simulink model "controlMCUSlugsMKIINewNav"  (Simulink 7.8)
settings: Solver=FixedStepDiscrete  SolverMode=SingleTasking  StartTime=0.0  StopTime=inf  FixedStep=0.01  RelTol=1e-3
InitFcn:
  | mcuInit
values from neighbouring files (symbols this model uses):
  apSampleTime = 0.01    [mcuInit.m]
  T = 0.01    [mcuInit.m]
undefined symbols (not defined in the file or in its folder): bda, bde, bdr, bdt, bICda, bICde, bICdr, bICdt, bpan, bPWMpan, bPWMtilt, broll, btilt, changeZoom, controlMCUInit, daTrimMax, daTrimMin, deTrimMax, deTrimMin, drTrimMax, drTrimMin, dtTrimMax, dtTrimMin, Function_Update, getAccBias, getAccels, getAttitude, getGSLocation, getISRLocation, getMidLevelCommands, getMobileLocation, getPassValues, getRangeOfParams, getRTB, getVned, getXYZ, gsRead, Init_onlyOnce, Init_Reset, mda, mde, mdr, mdt, mICda, mICde, mICdr, mICdt, mpan, mPWMpan, mPWMtilt, mroll, mtilt, PAR_CAM_X, PAR_CAM_Z, PAR_CONFIG_ROLL_R, PAR_CONFIG_YAW_R, PAR_L1_OMEGA, PAR_L1_ON_OFF, PAR_NAV_ISR_FAC, PAR_NAV_L2_BASE ... (+34)
libraries: dsPICdrivers x84, SLUGS_Library x12, simulink x7, aerolibobsolete x3, aerolibconvert2 x3, dspmtrx3 x1, aerolibtransform2 x1
(part 2 of 4)

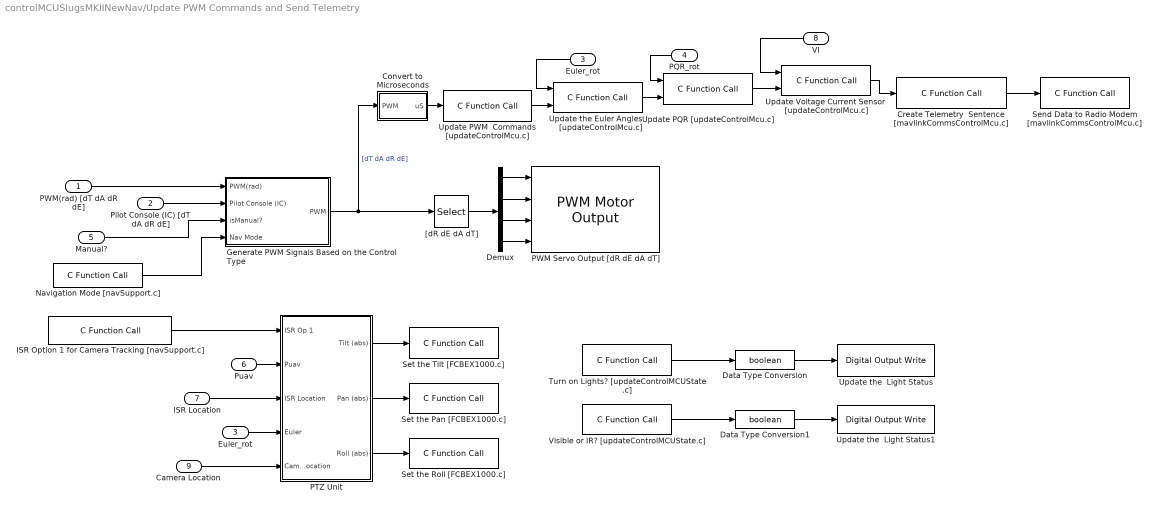
== system controlMCUSlugsMKIINewNav/Update PWM Commands and Send Telemetry ==
  PWM(rad) [dT dA dR dE] : Inport
  Pilot Console (IC) [dT dA dR dE] : Inport  Port=2
  Euler_rot : Inport  Port=3
  PQR_rot : Inport  Port=4
  Manual? : Inport  Port=5
  Puav : Inport  Port=6
  ISR Location : Inport  Port=7
  VI : Inport  Port=8
  Camera Location : Inport  Port=9
  Convert to Microseconds : Subsystem
  Create Telemetry  Sentence [mavlinkCommsControlMcu.c] : dsPICdrivers/OTHERS/C Function Call  Tag=dsPIC_dsPIC_CFunctionCall  FctUpdate=Output Function  fctName='prepareTelemetryMavlink'  INPUT_SIZE=1  INPUT1=--  INPUT2=--  INPUT3=--  OUTPUT_SIZE=120  OUTPUT1=uint8  SampleTime=.02  InputType=[ ]  OutputType=[ 2 ]  FctDeclaration=extern void prepareTelemetryMavlink(uint8_T* y1);  FctCall=prepareTelemetryMavlink(*%y1);  OrderingInOutPopup=Input  FctStart=None  FctStart_Name=Init_onlyOnce  FctStart_Declaration=inline extern void Init_onlyOnce();  FctStart_Call=Init_onlyOnce();  FctInit=None  FctInit_Name=Init_Reset  FctInit_Declaration=inline extern void Init_Reset();  FctInit_Call=Init_Reset();  PinDigitalInput=[]  PinDigitalOutput=[]  AnalogueInput=[]
  Data Type Conversion : DataTypeConversion  OutDataTypeStr=boolean
  Data Type Conversion1 : DataTypeConversion  OutDataTypeStr=boolean
  Demux : Demux
  "Euler_rot " : InportShadow  Port=3
  Generate PWM Signals Based on the Control Type : Subsystem
  ISR Option 1 for Camera Tracking [navSupport.c] : dsPICdrivers/OTHERS/C Function Call  Tag=dsPIC_dsPIC_CFunctionCall  FctUpdate=Output Function  fctName='getISRCameraOption1'  INPUT_SIZE=1  INPUT1=--  INPUT2=--  INPUT3=--  OUTPUT_SIZE=1  OUTPUT1=uint8  SampleTime=.01  InputType=[ ]  OutputType=[ 2 ]  FctDeclaration=extern uint8_T getISRCameraOption1();  FctCall=%y1 = getISRCameraOption1();  OrderingInOutPopup=None  FctStart=None  FctStart_Name=Init_onlyOnce  FctStart_Declaration=inline extern void Init_onlyOnce();  FctStart_Call=Init_onlyOnce();  FctInit=None  FctInit_Name=Init_Reset  FctInit_Declaration=inline extern void Init_Reset();  FctInit_Call=Init_Reset();  PinDigitalInput=[]  PinDigitalOutput=[]  AnalogueInput=[]
  Navigation Mode [navSupport.c] : dsPICdrivers/OTHERS/C Function Call  Tag=dsPIC_dsPIC_CFunctionCall  FctUpdate=Output Function  fctName='getNavMode'  INPUT_SIZE=1  INPUT1=--  INPUT2=--  INPUT3=--  OUTPUT_SIZE=1  OUTPUT1=uint8  SampleTime=.01  InputType=[ ]  OutputType=[ 2 ]  FctDeclaration=extern uint8_T getNavMode();  FctCall=%y1 = getNavMode();  OrderingInOutPopup=None  FctStart=None  FctStart_Name=Init_onlyOnce  FctStart_Declaration=inline extern void Init_onlyOnce();  FctStart_Call=Init_onlyOnce();  FctInit=None  FctInit_Name=Init_Reset  FctInit_Declaration=inline extern void Init_Reset();  FctInit_Call=Init_Reset();  PinDigitalInput=[]  PinDigitalOutput=[]  AnalogueInput=[]
  PTZ Unit : Subsystem
  PWM Servo Output [dR dE dA dT] : dsPICdrivers/Peripheral I//O/PWM Motor Output  Tag=dsPIC_PWM_Motor  Priority=5  PWMref=1  PWM12=1  InputEnableChk=off  InputPeriodeChk=off  Channel=[1 2 3 4]  TPeriode=.02  PrescalerValue=16  PeriodeInteger=25000  MaxName='PWM'  Centered=on  HChannelON=off  Info="Nbr Bits : 15.6096  ||  PWM = 50000  ||  Prescaler = 16"  Delay=0  IntPriority=5  nbrPwmChannelPIC=4  Status=OK  DeadTimePrescaleA=.0126*1e-3  DeadTimePrescaleB=0  DeadTimeInfo="Dead Time A = 1.26e-005  ||  Dead Time B = 0"  DTPWM1a=Prescaler A  DTPWM1i=Prescaler A  DTPWM2a=Prescaler A  DTPWM2i=Prescaler A  DTPWM3a=Prescaler A  DTPWM3i=Prescaler A  DTPWM4a=Prescaler A  DTPWM4i=Prescaler A  DTCON1=255  DTCON2=0  FAULTA_FLATM=Re-Enable PWM when Fault Pin is desactivated  FaultA_Output=off  FaultA_PWM1_State=No Changes (PWM)  FaultA_PWM2_State=No Changes (PWM)  FaultA_PWM3_State=No Changes (PWM)  FaultA_PWM4_State=No Changes (PWM)  OVDCON=off
  Send Data to Radio Modem [mavlinkCommsControlMcu.c] : dsPICdrivers/OTHERS/C Function Call  Tag=dsPIC_dsPIC_CFunctionCall  FctUpdate=Output Function  fctName='send2GS'  INPUT_SIZE=120  INPUT1=uint8  INPUT2=--  INPUT3=--  OUTPUT_SIZE=1  OUTPUT1=--  SampleTime=0.02  InputType=[ 2 ]  OutputType=[ ]  FctDeclaration=extern void send2GS(uint8_T* u1);  FctCall=send2GS(*%u1);  OrderingInOutPopup=None  FctStart=None  FctStart_Name=Init_onlyOnce  FctStart_Declaration=inline extern void Init_onlyOnce();  FctStart_Call=Init_onlyOnce();  FctInit=None  FctInit_Name=Init_Reset  FctInit_Declaration=inline extern void Init_Reset();  FctInit_Call=Init_Reset();  PinDigitalInput=[]  PinDigitalOutput=[]  AnalogueInput=[]
  Set the Pan [FCBEX1000.c] : dsPICdrivers/OTHERS/C Function Call  Tag=dsPIC_dsPIC_CFunctionCall  FctUpdate=Output Function  fctName='updatePan'  INPUT_SIZE=1  INPUT1=uint16  INPUT2=--  INPUT3=--  OUTPUT_SIZE=1  OUTPUT1=--  SampleTime=-1  InputType=[ 4 ]  OutputType=[ ]  FctDeclaration=extern void updatePan(uint16_T u1);  FctCall=updatePan(%u1);  OrderingInOutPopup=None  FctStart=None  FctStart_Name=Init_onlyOnce  FctStart_Declaration=inline extern void Init_onlyOnce();  FctStart_Call=Init_onlyOnce();  FctInit=None  FctInit_Name=Init_Reset  FctInit_Declaration=inline extern void Init_Reset();  FctInit_Call=Init_Reset();  PinDigitalInput=[]  PinDigitalOutput=[]  AnalogueInput=[]
  Set the Roll [FCBEX1000.c] : dsPICdrivers/OTHERS/C Function Call  Tag=dsPIC_dsPIC_CFunctionCall  FctUpdate=Output Function  fctName='updateRoll'  INPUT_SIZE=1  INPUT1=uint16  INPUT2=--  INPUT3=--  OUTPUT_SIZE=1  OUTPUT1=--  SampleTime=-1  InputType=[ 4 ]  OutputType=[ ]  FctDeclaration=extern void updateRoll(uint16_T u1);  FctCall=updateRoll(%u1);  OrderingInOutPopup=None  FctStart=None  FctStart_Name=Init_onlyOnce  FctStart_Declaration=inline extern void Init_onlyOnce();  FctStart_Call=Init_onlyOnce();  FctInit=None  FctInit_Name=Init_Reset  FctInit_Declaration=inline extern void Init_Reset();  FctInit_Call=Init_Reset();  PinDigitalInput=[]  PinDigitalOutput=[]  AnalogueInput=[]
  Set the Tilt [FCBEX1000.c] : dsPICdrivers/OTHERS/C Function Call  Tag=dsPIC_dsPIC_CFunctionCall  FctUpdate=Output Function  fctName='updateTilt'  INPUT_SIZE=1  INPUT1=uint16  INPUT2=--  INPUT3=--  OUTPUT_SIZE=1  OUTPUT1=--  SampleTime=-1  InputType=[ 4 ]  OutputType=[ ]  FctDeclaration=extern void updateTilt(uint16_T u1);  FctCall=updateTilt(%u1);  OrderingInOutPopup=None  FctStart=None  FctStart_Name=Init_onlyOnce  FctStart_Declaration=inline extern void Init_onlyOnce();  FctStart_Call=Init_onlyOnce();  FctInit=None  FctInit_Name=Init_Reset  FctInit_Declaration=inline extern void Init_Reset();  FctInit_Call=Init_Reset();  PinDigitalInput=[]  PinDigitalOutput=[]  AnalogueInput=[]
  Turn on Lights? [updateControlMCUState.c] : dsPICdrivers/OTHERS/C Function Call  Tag=dsPIC_dsPIC_CFunctionCall  FctUpdate=Output Function  fctName='getLightsOnOff'  INPUT_SIZE=1  INPUT1=--  INPUT2=--  INPUT3=--  OUTPUT_SIZE=1  OUTPUT1=uint8  SampleTime=0.01  InputType=[ ]  OutputType=[ 2 ]  FctDeclaration=extern uint8_T getLightsOnOff();  FctCall=%y1 = getLightsOnOff();  OrderingInOutPopup=None  FctStart=None  FctStart_Name=Init_onlyOnce  FctStart_Declaration=inline extern void Init_onlyOnce();  FctStart_Call=Init_onlyOnce();  FctInit=None  FctInit_Name=Init_Reset  FctInit_Declaration=inline extern void Init_Reset();  FctInit_Call=Init_Reset();  PinDigitalInput=[]  PinDigitalOutput=[]  AnalogueInput=[]
  "Update PQR [updateControlMcu.c] " : dsPICdrivers/OTHERS/C Function Call  Tag=dsPIC_dsPIC_CFunctionCall  FctUpdate=Output Function  fctName='updatePQR'  INPUT_SIZE=3  INPUT1=real32  INPUT2=--  INPUT3=--  OUTPUT_SIZE=1  OUTPUT1=--  SampleTime=.01  InputType=[ 7 ]  OutputType=[ ]  FctDeclaration=extern void updatePQR(real32_T* u1);  FctCall=updatePQR(*%u1);  OrderingInOutPopup=Input & Output  FctStart=None  FctStart_Name=Init_onlyOnce  FctStart_Declaration=inline extern void Init_onlyOnce();  FctStart_Call=Init_onlyOnce();  FctInit=None  FctInit_Name=Init_Reset  FctInit_Declaration=inline extern void Init_Reset();  FctInit_Call=Init_Reset();  PinDigitalInput=[]  PinDigitalOutput=[]  AnalogueInput=[]
  Update PWM  Commands [updateControlMcu.c] : dsPICdrivers/OTHERS/C Function Call  Tag=dsPIC_dsPIC_CFunctionCall  FctUpdate=Output Function  fctName='updatePWM'  INPUT_SIZE=4  INPUT1=uint16  INPUT2=--  INPUT3=--  OUTPUT_SIZE=1  OUTPUT1=--  SampleTime=-1  InputType=[ 4 ]  OutputType=[ ]  FctDeclaration=extern void updatePWM(uint16_T* u1);  FctCall=updatePWM(*%u1);  OrderingInOutPopup=Output  FctStart=None  FctStart_Name=Init_onlyOnce  FctStart_Declaration=inline extern void Init_onlyOnce();  FctStart_Call=Init_onlyOnce();  FctInit=None  FctInit_Name=Init_Reset  FctInit_Declaration=inline extern void Init_Reset();  FctInit_Call=Init_Reset();  PinDigitalInput=[]  PinDigitalOutput=[]  AnalogueInput=[]
  Update Voltage Current Sensor  [updateControlMcu.c] : dsPICdrivers/OTHERS/C Function Call  Tag=dsPIC_dsPIC_CFunctionCall  FctUpdate=Output Function  fctName='updateVISensor'  INPUT_SIZE=2  INPUT1=uint16  INPUT2=--  INPUT3=--  OUTPUT_SIZE=1  OUTPUT1=--  SampleTime=.01  InputType=[ 4 ]  OutputType=[ ]  FctDeclaration=extern void updateVISensor(uint16_T* u1);  FctCall=updateVISensor(*%u1);  OrderingInOutPopup=Input & Output  FctStart=None  FctStart_Name=Init_onlyOnce  FctStart_Declaration=inline extern void Init_onlyOnce();  FctStart_Call=Init_onlyOnce();  FctInit=None  FctInit_Name=Init_Reset  FctInit_Declaration=inline extern void Init_Reset();  FctInit_Call=Init_Reset();  PinDigitalInput=[]  PinDigitalOutput=[]  AnalogueInput=[]
  Update the  Light Status : dsPICdrivers/Digital I//O/Digital Output Write  Tag=dsPIC_Digital_Output  Priority=5  PORT=G  Pin=[15]  Simultaneous=off  OrderingInOutPopup=None
  Update the  Light Status1 : dsPICdrivers/Digital I//O/Digital Output Write  Tag=dsPIC_Digital_Output  Priority=5  PORT=G  Pin=[7]  Simultaneous=off  OrderingInOutPopup=None
  "Update the Euler Angles [updateControlMcu.c] " : dsPICdrivers/OTHERS/C Function Call  Tag=dsPIC_dsPIC_CFunctionCall  FctUpdate=Output Function  fctName='updateEuler'  INPUT_SIZE=3  INPUT1=real32  INPUT2=--  INPUT3=--  OUTPUT_SIZE=1  OUTPUT1=--  SampleTime=.01  InputType=[ 7 ]  OutputType=[ ]  FctDeclaration=extern void updateEuler(real32_T* u1);  FctCall=updateEuler(*%u1);  OrderingInOutPopup=Input & Output  FctStart=None  FctStart_Name=Init_onlyOnce  FctStart_Declaration=inline extern void Init_onlyOnce();  FctStart_Call=Init_onlyOnce();  FctInit=None  FctInit_Name=Init_Reset  FctInit_Declaration=inline extern void Init_Reset();  FctInit_Call=Init_Reset();  PinDigitalInput=[]  PinDigitalOutput=[]  AnalogueInput=[]
  Visible or IR? [updateControlMCUState.c] : dsPICdrivers/OTHERS/C Function Call  Tag=dsPIC_dsPIC_CFunctionCall  FctUpdate=Output Function  fctName='getLightsDayNight'  INPUT_SIZE=1  INPUT1=--  INPUT2=--  INPUT3=--  OUTPUT_SIZE=1  OUTPUT1=uint8  SampleTime=0.01  InputType=[ ]  OutputType=[ 2 ]  FctDeclaration=extern uint8_T getLightsDayNight();  FctCall=%y1 = getLightsDayNight();  OrderingInOutPopup=None  FctStart=None  FctStart_Name=Init_onlyOnce  FctStart_Declaration=inline extern void Init_onlyOnce();  FctStart_Call=Init_onlyOnce();  FctInit=None  FctInit_Name=Init_Reset  FctInit_Declaration=inline extern void Init_Reset();  FctInit_Call=Init_Reset();  PinDigitalInput=[]  PinDigitalOutput=[]  AnalogueInput=[]
  "[dR dE dA dT]" : Selector  InputPortWidth=4  IndexOptions=Index vector (dialog)  Indices=[3 4 2 1]  OutputSizes=1
  wires:
  Create Telemetry  Sentence [mavlinkCommsControlMcu.c]/1 -> Send Data to Radio Modem [mavlinkCommsControlMcu.c]/1
  Navigation Mode [navSupport.c]/1 -> Generate PWM Signals Based on the Control Type/4(Nav Mode)
  "[dR dE dA dT]"/1 -> Demux/1
  Demux/1 -> PWM Servo Output [dR dE dA dT]/1
  Demux/2 -> PWM Servo Output [dR dE dA dT]/2
  Demux/3 -> PWM Servo Output [dR dE dA dT]/3
  Demux/4 -> PWM Servo Output [dR dE dA dT]/4
  Generate PWM Signals Based on the Control Type/1(PWM) -> "[dR dE dA dT]"/1, Convert to Microseconds/1(PWM)  "[dT dA dR dE]"
  PWM(rad) [dT dA dR dE]/1 -> Generate PWM Signals Based on the Control Type/1(PWM(rad))
  Pilot Console (IC) [dT dA dR dE]/1 -> Generate PWM Signals Based on the Control Type/2(Pilot Console (IC))
  Euler_rot/1 -> "Update the Euler Angles [updateControlMcu.c] "/1
  PQR_rot/1 -> "Update PQR [updateControlMcu.c] "/1
  Update PWM  Commands [updateControlMcu.c]/1 -> "Update the Euler Angles [updateControlMcu.c] "/2
  "Update the Euler Angles [updateControlMcu.c] "/1 -> "Update PQR [updateControlMcu.c] "/2
  Convert to Microseconds/1(uS) -> Update PWM  Commands [updateControlMcu.c]/1
  Manual?/1 -> Generate PWM Signals Based on the Control Type/3(isManual?)
  PTZ Unit/2(Pan (abs)) -> Set the Pan [FCBEX1000.c]/1
  PTZ Unit/1(Tilt (abs)) -> Set the Tilt [FCBEX1000.c]/1
  ISR Option 1 for Camera Tracking [navSupport.c]/1 -> PTZ Unit/1(ISR Op 1)
  Puav/1 -> PTZ Unit/2(Puav)
  ISR Location/1 -> PTZ Unit/3(ISR Location)
  "Euler_rot "/1 -> PTZ Unit/4(Euler)
  PTZ Unit/3(Roll (abs)) -> Set the Roll [FCBEX1000.c]/1
  Turn on Lights? [updateControlMCUState.c]/1 -> Data Type Conversion/1
  Visible or IR? [updateControlMCUState.c]/1 -> Data Type Conversion1/1
  Data Type Conversion/1 -> Update the  Light Status/1
  Data Type Conversion1/1 -> Update the  Light Status1/1
  "Update PQR [updateControlMcu.c] "/1 -> Update Voltage Current Sensor  [updateControlMcu.c]/2
  Update Voltage Current Sensor  [updateControlMcu.c]/1 -> Create Telemetry  Sentence [mavlinkCommsControlMcu.c]/1
  VI/1 -> Update Voltage Current Sensor  [updateControlMcu.c]/1
  Camera Location/1 -> PTZ Unit/5(Camera Location)

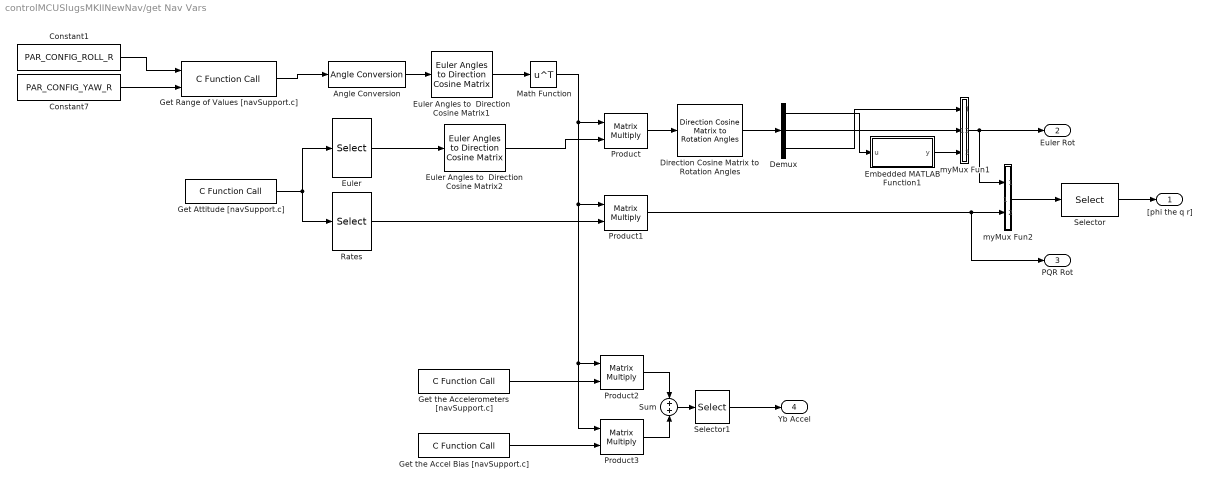
== system controlMCUSlugsMKIINewNav/get Nav Vars ==
  Angle Conversion : aerolibconvert2/Angle Conversion  IU=deg  OU=rad
  Constant1 : Constant  Value=PAR_CONFIG_ROLL_R  OutDataTypeStr=uint8
  Constant7 : Constant  Value=PAR_CONFIG_YAW_R  OutDataTypeStr=uint8
  Demux : Demux  Outputs=3
  Direction Cosine Matrix to Rotation Angles : aerolibtransform2/Direction Cosine Matrix to Rotation Angles  rotationOrder=ZYX  lim=Default
      settings: AttributesFormatString=Rotation Order: %<rotationOrder>
  Embedded MATLAB Function1 : MATLAB Function  TreatAsAtomicUnit=on
  Euler : Selector  InputPortWidth=6  IndexOptions=Index vector (dialog)  Indices=[1 2 3]  OutputSizes=1
  Euler Angles to  Direction Cosine Matrix1 : aerolibobsolete/Euler Angles to  Direction Cosine Matrix
  Euler Angles to  Direction Cosine Matrix2 : aerolibobsolete/Euler Angles to  Direction Cosine Matrix
  Get Attitude [navSupport.c] : dsPICdrivers/OTHERS/C Function Call  Tag=dsPIC_dsPIC_CFunctionCall  FctUpdate=Output Function  fctName='getAttitude'  INPUT_SIZE=1  INPUT1=--  INPUT2=--  INPUT3=--  OUTPUT_SIZE=6  OUTPUT1=real32  SampleTime=.01  InputType=[ ]  OutputType=[ 7 ]  FctDeclaration=extern void getAttitude(real32_T* y1);  FctCall=getAttitude(*%y1);  OrderingInOutPopup=None  FctStart=None  FctStart_Name=Init_onlyOnce  FctStart_Declaration=inline extern void Init_onlyOnce();  FctStart_Call=Init_onlyOnce();  FctInit=None  FctInit_Name=Init_Reset  FctInit_Declaration=inline extern void Init_Reset();  FctInit_Call=Init_Reset();  PinDigitalInput=[]  PinDigitalOutput=[]  AnalogueInput=[]
  Get Range of Values [navSupport.c] : dsPICdrivers/OTHERS/C Function Call  Tag=dsPIC_dsPIC_CFunctionCall  FctUpdate=Output Function  fctName='getRangeOfParams'  INPUT_SIZE=1  INPUT1=uint8  INPUT2=uint8  INPUT3=--  OUTPUT_SIZE=3  OUTPUT1=real32  SampleTime=.01  InputType=[ 2 2 ]  OutputType=[ 7 ]  FctDeclaration=extern void getRangeOfParams(uint8_T u1, uint8_T u2,real32_T* y1);  FctCall=getRangeOfParams(%u1, %u2, *%y1);  OrderingInOutPopup=None  FctStart=None  FctStart_Name=Init_onlyOnce  FctStart_Declaration=inline extern void Init_onlyOnce();  FctStart_Call=Init_onlyOnce();  FctInit=None  FctInit_Name=Init_Reset  FctInit_Declaration=inline extern void Init_Reset();  FctInit_Call=Init_Reset();  PinDigitalInput=[]  PinDigitalOutput=[]  AnalogueInput=[]
  Get the Accel Bias [navSupport.c] : dsPICdrivers/OTHERS/C Function Call  Tag=dsPIC_dsPIC_CFunctionCall  FctUpdate=Output Function  fctName='getAccBias'  INPUT_SIZE=1  INPUT1=--  INPUT2=--  INPUT3=--  OUTPUT_SIZE=3  OUTPUT1=real32  SampleTime=.01  InputType=[ ]  OutputType=[ 7 ]  FctDeclaration=extern void getAccBias(real32_T* y1);  FctCall=getAccBias(*%y1);  OrderingInOutPopup=None  FctStart=None  FctStart_Name=Init_onlyOnce  FctStart_Declaration=inline extern void Init_onlyOnce();  FctStart_Call=Init_onlyOnce();  FctInit=None  FctInit_Name=Init_Reset  FctInit_Declaration=inline extern void Init_Reset();  FctInit_Call=Init_Reset();  PinDigitalInput=[]  PinDigitalOutput=[]  AnalogueInput=[]
  Get the Accelerometers [navSupport.c] : dsPICdrivers/OTHERS/C Function Call  Tag=dsPIC_dsPIC_CFunctionCall  FctUpdate=Output Function  fctName='getAccels'  INPUT_SIZE=1  INPUT1=--  INPUT2=--  INPUT3=--  OUTPUT_SIZE=3  OUTPUT1=real32  SampleTime=.01  InputType=[ ]  OutputType=[ 7 ]  FctDeclaration=extern void getAccels(real32_T* y1);  FctCall=getAccels(*%y1);  OrderingInOutPopup=None  FctStart=None  FctStart_Name=Init_onlyOnce  FctStart_Declaration=inline extern void Init_onlyOnce();  FctStart_Call=Init_onlyOnce();  FctInit=None  FctInit_Name=Init_Reset  FctInit_Declaration=inline extern void Init_Reset();  FctInit_Call=Init_Reset();  PinDigitalInput=[]  PinDigitalOutput=[]  AnalogueInput=[]
  Math Function : Math  Operator=transpose  SaturateOnIntegerOverflow=on
  Product{,1..3} (4 alike) : Product  Multiplication=Matrix(*)  RndMeth=Zero
  Rates : Selector  InputPortWidth=6  IndexOptions=Index vector (dialog)  Indices=[4 5 6]  OutputSizes=1
  Selector : Selector  InputPortWidth=6  IndexOptions=Index vector (dialog)  Indices=[1 2 5 6]  OutputSizes=1
  Selector1 : Selector  InputPortWidth=3  IndexOptions=Index vector (dialog)  Indices=[2]  OutputSizes=1
  Sum : Sum  Inputs=+|+
  myMux Fun1 : MATLAB Function  TreatAsAtomicUnit=on
  myMux Fun2 : MATLAB Function  TreatAsAtomicUnit=on
  "[phi the q r]" : Outport
  Euler Rot : Outport  Port=2
  PQR Rot : Outport  Port=3
  Yb Accel : Outport  Port=4
  wires:
  Selector/1 -> "[phi the q r]"/1
  Get Attitude [navSupport.c]/1 -> Euler/1, Rates/1
  Euler/1 -> Euler Angles to  Direction Cosine Matrix2/1
  Euler Angles to  Direction Cosine Matrix2/1 -> Product/2
  Euler Angles to  Direction Cosine Matrix1/1 -> Math Function/1
  Angle Conversion/1 -> Euler Angles to  Direction Cosine Matrix1/1
  Product/1 -> Direction Cosine Matrix to Rotation Angles/1
  Rates/1 -> Product1/2
  myMux Fun1/1(y) -> Euler Rot/1, myMux Fun2/1(u1)
  Product1/1 -> myMux Fun2/2(u2), PQR Rot/1
  myMux Fun2/1(y) -> Selector/1
  Math Function/1 -> Product/1, Product1/1, Product2/1, Product3/1
  Get the Accelerometers [navSupport.c]/1 -> Product2/2
  Get the Accel Bias [navSupport.c]/1 -> Product3/2
  Product2/1 -> Sum/1
  Product3/1 -> Sum/2
  Sum/1 -> Selector1/1
  Selector1/1 -> Yb Accel/1
  Constant1/1 -> Get Range of Values [navSupport.c]/1
  Constant7/1 -> Get Range of Values [navSupport.c]/2
  Get Range of Values [navSupport.c]/1 -> Angle Conversion/1
  Demux/1 -> Embedded MATLAB Function1/1(u)
  Direction Cosine Matrix to Rotation Angles/1 -> Demux/1
  Demux/2 -> myMux Fun1/2(u2)
  Demux/3 -> myMux Fun1/1(u1)
  Embedded MATLAB Function1/1(y) -> myMux Fun1/3(u3)

== system controlMCUSlugsMKIINewNav/Data  Sources/Compute Load ==
  Calculus Time Step : dsPICdrivers/OTHERS/Calculus Time Step  Tag=dsPIC_CalculusTimeStep  SampleTime=0.01  PR1chk=on
  Data Type Conversion12 : DataTypeConversion  OutDataTypeStr=uint8
  Data Type Conversion3 : DataTypeConversion  OutDataTypeStr=single
  Data Type Conversion4 : DataTypeConversion  OutDataTypeStr=single
  Divide : Product  Inputs=*/  OutDataTypeStr=double
  Gain : Gain  Gain=100
  Rounding Function : Rounding
  Load (%) : Outport
  wires:
  Calculus Time Step/1 -> Data Type Conversion4/1
  Calculus Time Step/2 -> Data Type Conversion3/1
  Divide/1 -> Gain/1
  Rounding Function/1 -> Data Type Conversion12/1
  Data Type Conversion3/1 -> Divide/2
  Data Type Conversion4/1 -> Divide/1
  Data Type Conversion12/1 -> Load (%)/1
  Gain/1 -> Rounding Function/1

== system controlMCUSlugsMKIINewNav/Inner Loop/ Navigation/Compute psi_dot_m ==
  r_m : Inport
  phi_m : Inport  Port=2
  q_m : Inport  Port=3
  Product : Product  SampleTime=apSampleTime  RndMeth=Zero
  Product1 : Product  SampleTime=apSampleTime  RndMeth=Zero
  Protect NaNs : Subsystem
  Subtract : Sum  Inputs=2
  dsPIC_cos : SLUGS_Library/dsPIC_cos
  dsPIC_sin : SLUGS_Library/dsPIC_sin
  psi_dot_m : Outport
  wires:
  q_m/1 -> Product1/1
  Subtract/1 -> Protect NaNs/1(In1)
  phi_m/1 -> dsPIC_sin/1, dsPIC_cos/1
  r_m/1 -> Product/1
  Product1/1 -> Subtract/2
  Product/1 -> Subtract/1
  dsPIC_sin/1 -> Product1/2
  dsPIC_cos/1 -> Product/2
  Protect NaNs/1(Out1) -> psi_dot_m/1

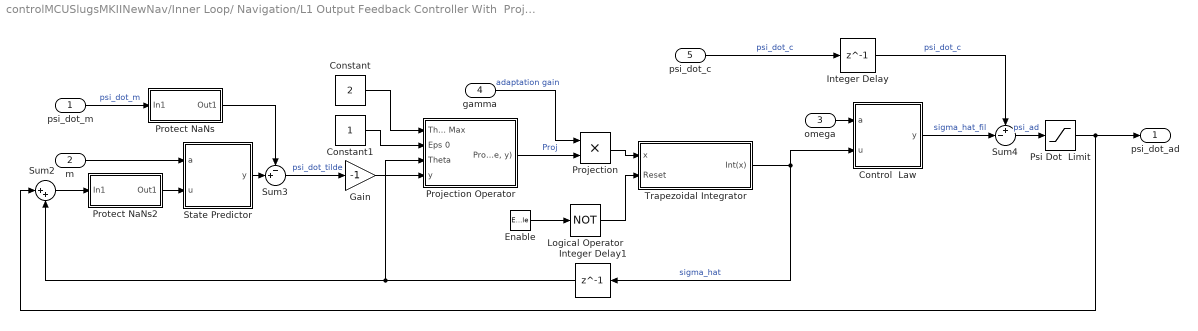
== system controlMCUSlugsMKIINewNav/Inner Loop/ Navigation/L1 Output Feedback Controller With  Projection Operator ==
  psi_dot_m : Inport
  m : Inport  Port=2
  omega : Inport  Port=3
  gamma : Inport  Port=4
  psi_dot_c : Inport  Port=5
  Enable : EnablePort  StatesWhenEnabling=reset  ShowOutputPort=on
  Constant : Constant  Value=2  OutDataTypeStr=single
  Constant1 : Constant  OutDataTypeStr=single
  Control  Law : Subsystem
      mask Display:
      | droots([],'-a','a')
      | port_label('input',1,'a')
      | port_label('input',2,'u')
      | port_label('output',1,'y')
  Gain : Gain  Gain=-1  OutDataTypeStr=Inherit: Same as input
  Integer Delay : Delay  DelayLength=1  InputProcessing=Inherited  SampleTime=.01
  Integer Delay1 : Delay  DelayLength=1  InputProcessing=Inherited  SampleTime=.01
  Logical Operator : Logic  Operator=NOT  AllPortsSameDT=off  OutDataTypeStr=uint(8)
  Projection : Product  OutDataTypeStr=single  SampleTime=apSampleTime  RndMeth=Zero
  Projection Operator : Subsystem
  Protect NaNs : Subsystem
  Protect NaNs2 : Subsystem
  Psi Dot  Limit : Saturate  UpperLimit=1  LowerLimit=-1  SampleTime=apSampleTime
  State Predictor : Subsystem
      mask Display:
      | droots([],'-a','a')
      | port_label('input',1,'a')
      | port_label('input',2,'u')
      | port_label('output',1,'y')
  Sum2 : Sum  Inputs=|++  OutDataTypeStr=single  SampleTime=apSampleTime
  Sum3 : Sum  Inputs=-+|  OutDataTypeStr=single  SampleTime=apSampleTime
  Sum4 : Sum  Inputs=+-|  OutDataTypeStr=single  SampleTime=apSampleTime
  Trapezoidal Integrator : Subsystem  AncestorBlock=SLUGS_Library/Control Blocks/PID Controller w//Anti-Windup/Trapezoidal Integrator  mask{T=apSampleTime, upperLimit=2, lowerLimit=-2}
      mask prompts: T "Sample Time"; upperLimit "Upper Saturation"; lowerLimit "Lower Saturation"
  psi_dot_ad : Outport
  wires:
  Integer Delay/1 -> Sum4/1  "psi_dot_c"
  State Predictor/1(y) -> Sum3/2
  Gain/1 -> Projection Operator/4(y)
  m/1 -> State Predictor/1(a)
  Sum2/1 -> Protect NaNs2/1(In1)
  psi_dot_m/1 -> Protect NaNs/1(In1)  "psi_dot_m"
  Sum3/1 -> Gain/1  "psi_dot_tilde"
  gamma/1 -> Projection/1  "adaptation gain"
  Projection/1 -> Trapezoidal Integrator/1(x)
  psi_dot_c/1 -> Integer Delay/1  "psi_dot_c"
  omega/1 -> Control  Law/1(a)
  Control  Law/1(y) -> Sum4/2  "sigma_hat_fil"
  Sum4/1 -> Psi Dot  Limit/1  "psi_ad"
  Projection Operator/1("Proj(the, y)") -> Projection/2  "Proj"
  Constant/1 -> Projection Operator/1(Theta Max)
  Constant1/1 -> Projection Operator/2(Eps 0)
  Integer Delay1/1 -> Sum2/2, Projection Operator/3(Theta)
  Enable/1 -> Logical Operator/1
  Logical Operator/1 -> Trapezoidal Integrator/2(Reset)
  Trapezoidal Integrator/1(Int(x)) -> Control  Law/2(u), Integer Delay1/1  "sigma_hat"
  Protect NaNs2/1(Out1) -> State Predictor/2(u)
  Protect NaNs/1(Out1) -> Sum3/1
  Psi Dot  Limit/1 -> psi_dot_ad/1, Sum2/1

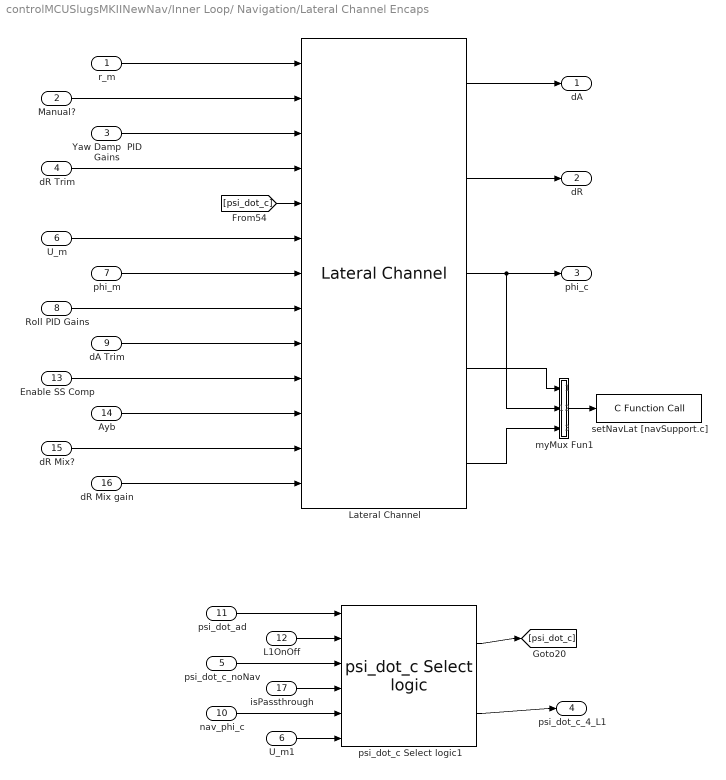
== system controlMCUSlugsMKIINewNav/Inner Loop/ Navigation/Lateral Channel Encaps ==
  r_m : Inport
  Manual? : Inport  Port=2
  Yaw Damp  PID Gains : Inport  Port=3
  dR Trim : Inport  Port=4
  psi_dot_c_noNav : Inport  Port=5
  U_m : Inport  Port=6
  phi_m : Inport  Port=7
  Roll PID Gains : Inport  Port=8
  dA Trim : Inport  Port=9
  nav_phi_c : Inport  Port=10
  psi_dot_ad : Inport  Port=11  SampleTime=apSampleTime
  L1OnOff : Inport  Port=12
  Enable SS Comp : Inport  Port=13
  Ayb : Inport  Port=14
  dR Mix? : Inport  Port=15
  dR Mix gain : Inport  Port=16
  isPassthrough : Inport  Port=17
  Lateral Channel : SLUGS_Library/Control Blocks/Lateral Channel
  U_m1 : InportShadow  Port=6
  myMux Fun1 : MATLAB Function  TreatAsAtomicUnit=on
  psi_dot_c Select logic1 : SLUGS_Library/Control Blocks/psi_dot_c Select logic
  setNavLat [navSupport.c] : dsPICdrivers/OTHERS/C Function Call  Tag=dsPIC_dsPIC_CFunctionCall  FctUpdate=Output Function  fctName='setNavLat'  INPUT_SIZE=3  INPUT1=real32  INPUT2=--  INPUT3=--  OUTPUT_SIZE=1  OUTPUT1=--  SampleTime=.01  InputType=[ 7 ]  OutputType=[ ]  FctDeclaration=extern void setNavLat(real32_T* u1);  FctCall=setNavLat(*%u1);  OrderingInOutPopup=None  FctStart=None  FctStart_Name=Init_onlyOnce  FctStart_Declaration=inline extern void Init_onlyOnce();  FctStart_Call=Init_onlyOnce();  FctInit=None  FctInit_Name=Init_Reset  FctInit_Declaration=inline extern void Init_Reset();  FctInit_Call=Init_Reset();  PinDigitalInput=[]  PinDigitalOutput=[]  AnalogueInput=[]
  dA : Outport
  dR : Outport  Port=2
  phi_c : Outport  Port=3
  psi_dot_c_4_L1 : Outport  Port=4
  wires:
  myMux Fun1/1(y) -> setNavLat [navSupport.c]/1
  Lateral Channel/4 -> myMux Fun1/1(u1)
  Lateral Channel/5 -> myMux Fun1/3(u3)
  dR Trim/1 -> Lateral Channel/4
  phi_m/1 -> Lateral Channel/7
  r_m/1 -> Lateral Channel/1
  Lateral Channel/1 -> dA/1
  Roll PID Gains/1 -> Lateral Channel/8
  dA Trim/1 -> Lateral Channel/9
  Enable SS Comp/1 -> Lateral Channel/10
  Manual?/1 -> Lateral Channel/2
  Ayb/1 -> Lateral Channel/11
  dR Mix gain/1 -> Lateral Channel/13
  Lateral Channel/2 -> dR/1
  Yaw Damp  PID Gains/1 -> Lateral Channel/3
  dR Mix?/1 -> Lateral Channel/12
  Lateral Channel/3 -> phi_c/1, myMux Fun1/2(u2)
  U_m/1 -> Lateral Channel/6
  nav_phi_c/1 -> psi_dot_c Select logic1/5
  U_m1/1 -> psi_dot_c Select logic1/6
  psi_dot_ad/1 -> psi_dot_c Select logic1/1
  L1OnOff/1 -> psi_dot_c Select logic1/2
  psi_dot_c_noNav/1 -> psi_dot_c Select logic1/3
  [psi_dot_c] -> Lateral Channel/5
  psi_dot_c Select logic1/1 -> [psi_dot_c]
  psi_dot_c Select logic1/2 -> psi_dot_c_4_L1/1
  isPassthrough/1 -> psi_dot_c Select logic1/4

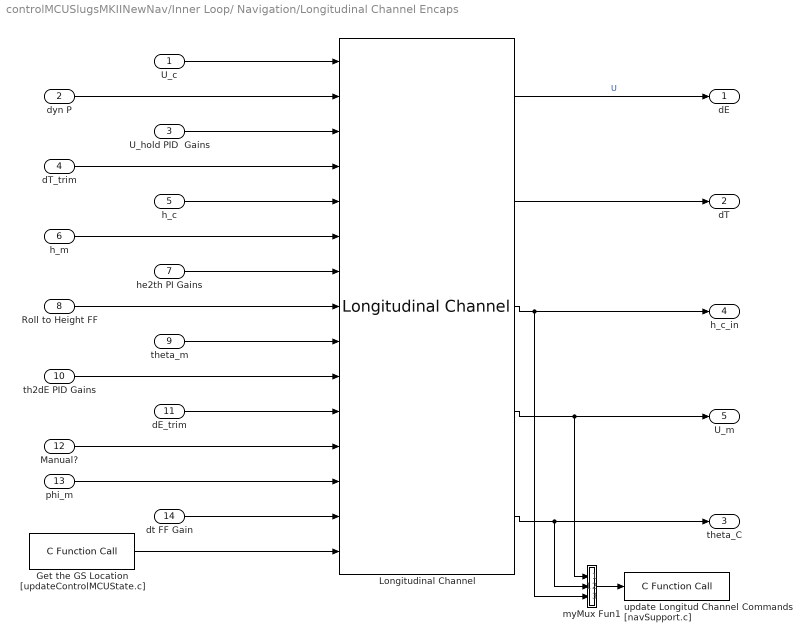
== system controlMCUSlugsMKIINewNav/Inner Loop/ Navigation/Longitudinal Channel Encaps ==
  U_c : Inport
  dyn P : Inport  Port=2
  U_hold PID  Gains : Inport  Port=3
  dT_trim : Inport  Port=4
  h_c : Inport  Port=5
  h_m : Inport  Port=6
  he2th PI Gains : Inport  Port=7
  Roll to Height FF : Inport  Port=8
  theta_m : Inport  Port=9
  th2dE PID Gains : Inport  Port=10
  dE_trim : Inport  Port=11
  Manual? : Inport  Port=12
  phi_m : Inport  Port=13
  dt FF Gain : Inport  Port=14
  Get the GS Location [updateControlMCUState.c] : dsPICdrivers/OTHERS/C Function Call  Tag=dsPIC_dsPIC_CFunctionCall  FctUpdate=Output Function  fctName='getGSLocation'  INPUT_SIZE=1  INPUT1=--  INPUT2=--  INPUT3=--  OUTPUT_SIZE=3  OUTPUT1=real32  SampleTime=0.01  InputType=[ ]  OutputType=[ 7 ]  FctDeclaration=extern void getGSLocation(real32_T* y1);  FctCall=getGSLocation(*%y1);  OrderingInOutPopup=None  FctStart=None  FctStart_Name=Init_onlyOnce  FctStart_Declaration=inline extern void Init_onlyOnce();  FctStart_Call=Init_onlyOnce();  FctInit=None  FctInit_Name=Init_Reset  FctInit_Declaration=inline extern void Init_Reset();  FctInit_Call=Init_Reset();  PinDigitalInput=[]  PinDigitalOutput=[]  AnalogueInput=[]
  Longitudinal Channel : SLUGS_Library/Control Blocks/Longitudinal Channel
  myMux Fun1 : MATLAB Function  TreatAsAtomicUnit=on
  update Longitud Channel Commands [navSupport.c] : dsPICdrivers/OTHERS/C Function Call  Tag=dsPIC_dsPIC_CFunctionCall  FctUpdate=Output Function  fctName='setNavLong'  INPUT_SIZE=3  INPUT1=real32  INPUT2=--  INPUT3=--  OUTPUT_SIZE=1  OUTPUT1=--  SampleTime=.01  InputType=[ 7 ]  OutputType=[ ]  FctDeclaration=extern void setNavLong(real32_T* u1);  FctCall=setNavLong(*%u1);  OrderingInOutPopup=None  FctStart=None  FctStart_Name=Init_onlyOnce  FctStart_Declaration=inline extern void Init_onlyOnce();  FctStart_Call=Init_onlyOnce();  FctInit=None  FctInit_Name=Init_Reset  FctInit_Declaration=inline extern void Init_Reset();  FctInit_Call=Init_Reset();  PinDigitalInput=[]  PinDigitalOutput=[]  AnalogueInput=[]
  dE : Outport
  dT : Outport  Port=2
  theta_C : Outport  Port=3
  h_c_in : Outport  Port=4
  U_m : Outport  Port=5
  wires:
  myMux Fun1/1(y) -> update Longitud Channel Commands [navSupport.c]/1
  U_c/1 -> Longitudinal Channel/1
  dyn P/1 -> Longitudinal Channel/2
  U_hold PID  Gains/1 -> Longitudinal Channel/3
  dT_trim/1 -> Longitudinal Channel/4
  h_m/1 -> Longitudinal Channel/6
  theta_m/1 -> Longitudinal Channel/9
  dE_trim/1 -> Longitudinal Channel/11
  Manual?/1 -> Longitudinal Channel/12
  he2th PI Gains/1 -> Longitudinal Channel/7
  Roll to Height FF/1 -> Longitudinal Channel/8
  th2dE PID Gains/1 -> Longitudinal Channel/10
  dt FF Gain/1 -> Longitudinal Channel/14
  h_c/1 -> Longitudinal Channel/5
  phi_m/1 -> Longitudinal Channel/13
  Get the GS Location [updateControlMCUState.c]/1 -> Longitudinal Channel/15
  Longitudinal Channel/1 -> dE/1  "U"
  Longitudinal Channel/2 -> dT/1
  Longitudinal Channel/3 -> h_c_in/1, myMux Fun1/3(u3)
  Longitudinal Channel/4 -> U_m/1, myMux Fun1/1(u1)
  Longitudinal Channel/5 -> theta_C/1, myMux Fun1/2(u2)

== system controlMCUSlugsMKIINewNav/Inner Loop/ Navigation/Navigation Encaps ==
  Puav : Inport  SampleTime=apSampleTime
  Max WP Idx : Inport  Port=2
  Vxyz : Inport  Port=3  SampleTime=apSampleTime
  T*(m) : Inport  Port=4
  U_c : Inport  Port=5
  WPFly : Inport  Port=6
  TurnLeadTime : Inport  Port=7
  RTB : Inport  Port=8
  Mobile Location : Inport  Port=9
  Follow Mobile? : Inport  Port=10
  MidLvl h_c : Inport  Port=11
  isApManual? : Inport  Port=12
  ISR Scale : Inport  Port=13
  Get ISR Location [navSupport.c] : dsPICdrivers/OTHERS/C Function Call  Tag=dsPIC_dsPIC_CFunctionCall  FctUpdate=Output Function  fctName='getISRLocation'  INPUT_SIZE=1  INPUT1=--  INPUT2=--  INPUT3=--  OUTPUT_SIZE=3  OUTPUT1=real32  SampleTime=.01  InputType=[ ]  OutputType=[ 7 ]  FctDeclaration=extern void getISRLocation(real32_T* y1);  FctCall=getISRLocation(*%y1);  OrderingInOutPopup=None  FctStart=None  FctStart_Name=Init_onlyOnce  FctStart_Declaration=inline extern void Init_onlyOnce();  FctStart_Call=Init_onlyOnce();  FctInit=None  FctInit_Name=Init_Reset  FctInit_Declaration=inline extern void Init_Reset();  FctInit_Call=Init_Reset();  PinDigitalInput=[]  PinDigitalOutput=[]  AnalogueInput=[]
  Navigation : SLUGS_Library/Navigation/Navigation
  Navigation Mode [navSupport.c] : dsPICdrivers/OTHERS/C Function Call  Tag=dsPIC_dsPIC_CFunctionCall  FctUpdate=Output Function  fctName='getNavMode'  INPUT_SIZE=1  INPUT1=--  INPUT2=--  INPUT3=--  OUTPUT_SIZE=1  OUTPUT1=uint8  SampleTime=.01  InputType=[ ]  OutputType=[ 2 ]  FctDeclaration=extern uint8_T getNavMode();  FctCall=%y1 = getNavMode();  OrderingInOutPopup=None  FctStart=None  FctStart_Name=Init_onlyOnce  FctStart_Declaration=inline extern void Init_onlyOnce();  FctStart_Call=Init_onlyOnce();  FctInit=None  FctInit_Name=Init_Reset  FctInit_Declaration=inline extern void Init_Reset();  FctInit_Call=Init_Reset();  PinDigitalInput=[]  PinDigitalOutput=[]  AnalogueInput=[]
  h_c : Outport
  phi_c : Outport  Port=2
  ISR Loc : Outport  Port=3
  "Puav " : Outport  Port=4
  wires:
  Navigation Mode [navSupport.c]/1 -> Navigation/1
  T*(m)/1 -> Navigation/2
  WPFly/1 -> Navigation/3
  RTB/1 -> Navigation/4
  isApManual?/1 -> Navigation/5
  Navigation/1 -> h_c/1
  Navigation/2 -> phi_c/1
  Puav/1 -> Navigation/6
  Navigation/4 -> "Puav "/1
  Get ISR Location [navSupport.c]/1 -> Navigation/7
  Max WP Idx/1 -> Navigation/8
  Vxyz/1 -> Navigation/9
  U_c/1 -> Navigation/10
  TurnLeadTime/1 -> Navigation/11
  Mobile Location/1 -> Navigation/12
  Follow Mobile?/1 -> Navigation/13
  MidLvl h_c/1 -> Navigation/14
  ISR Scale/1 -> Navigation/15
  Navigation/3 -> ISR Loc/1

== system controlMCUSlugsMKIINewNav/Inner Loop/ Navigation/Protect NaNs ==
  In1 : Inport
  Integer Delay3 : Delay  DelayLength=1  InputProcessing=Inherited  SampleTime=T
  Relational Operator2 : RelationalOperator  Operator===  OutDataTypeStr=uint(8)
  Switch3 : Switch  Criteria=u2 > Threshold  Threshold=0.3  SampleTime=.01
  Out1 : Outport
  wires:
  Integer Delay3/1 -> Switch3/3
  Switch3/1 -> Out1/1, Integer Delay3/1
  In1/1 -> Relational Operator2/2, Relational Operator2/1, Switch3/1
  Relational Operator2/1 -> Switch3/2

== system controlMCUSlugsMKIINewNav/Trim Vals/Bufffer IC ==
  Pilot Console : Inport
  Buffer IC Channel : MATLAB Function  TreatAsAtomicUnit=on
  Buffer IC Channel1 : MATLAB Function  TreatAsAtomicUnit=on
  Buffer IC Channel2 : MATLAB Function  TreatAsAtomicUnit=on
  Buffer IC Channel3 : MATLAB Function  TreatAsAtomicUnit=on
  Demux : Demux
  dT_buf : Outport
  dA_buf : Outport  Port=2
  dR_buf : Outport  Port=3
  dE_buf : Outport  Port=4
  wires:
  Demux/1 -> Buffer IC Channel/1(latest)
  Demux/2 -> Buffer IC Channel1/1(latest)
  Demux/3 -> Buffer IC Channel2/1(latest)
  Demux/4 -> Buffer IC Channel3/1(latest)
  Pilot Console/1 -> Demux/1
  Buffer IC Channel/1(history) -> dT_buf/1
  Buffer IC Channel1/1(history) -> dA_buf/1
  Buffer IC Channel2/1(history) -> dR_buf/1
  Buffer IC Channel3/1(history) -> dE_buf/1

== system controlMCUSlugsMKIINewNav/Trim Vals/Control Surface Input ==
  2 sec  tau : Subsystem  mask(Tustin1stOrderLowpassAutoInitialCondition){f=0.1, T=T}
      mask prompts: f "Lowpass Frequency"; T "Sample Time"
      mask help: Takes a 3db rolloff frequency (in Hz, NOT radians/s) and a sample time. Performs a symbolic Tustin conversion and implements in a discrete filter. The initial output of the filter is set by the first sample.
      mask Help: Enter the desired 3db rolloff frequency in Hz and the sample time. Initial conditions are sampled automatically.
      mask Display: fprintf('%.2f Hz lowpass',f)
  2 sec  tau1 : Subsystem  mask(Tustin1stOrderLowpassAutoInitialCondition){f=0.1, T=T}
      mask prompts: f "Lowpass Frequency"; T "Sample Time"
      mask help: Takes a 3db rolloff frequency (in Hz, NOT radians/s) and a sample time. Performs a symbolic Tustin conversion and implements in a discrete filter. The initial output of the filter is set by the first sample.
      mask Help: Enter the desired 3db rolloff frequency in Hz and the sample time. Initial conditions are sampled automatically.
      mask Display: fprintf('%.2f Hz lowpass',f)
  Data Type Conversion1 : DataTypeConversion  OutDataTypeStr=uint16
  Data Type Conversion2 : DataTypeConversion  OutDataTypeStr=single
  Data Type Conversion3 : DataTypeConversion  OutDataTypeStr=single
  Data Type Conversion4 : DataTypeConversion  OutDataTypeStr=uint16
  Input Capture : dsPICdrivers/Peripheral I//O/Input Capture  Tag=dsPIC_PWM_IC  Priority=5  IntPriority=6  Channel=[ 1 2 3 4 5 7 8]  Channel_UP_Down_Periode="[1  1  1  1  1  1  1]"  MaxChannel="[0.0025      0.0025      0.0025      0.0025      0.0025      0.0025      0.0025]"  SafeMarge="[10  10  10  10  10  10  10]"  MaxName=' IC1max , IC2max , IC3max , IC4max , IC5max , IC7max , IC8max '  Precision="[13.6094      13.6094      13.6094      13.6094      13.6094      13.6094      13.6094]"  Timer="[2  2  2  2  2  2  2]"  ChangeDetected="[0  0  0  0  0  0  0]"  ChangeDetectedPortRef=3  SampleTime=.01  Status=OK
  myMux Fun1 : MATLAB Function  TreatAsAtomicUnit=on
  myMux Fun5 : MATLAB Function  TreatAsAtomicUnit=on
  Pilot Console : Outport
  Voltage/Current Sensor : Outport  Port=2
  wires:
  myMux Fun5/1(y) -> Pilot Console/1
  Input Capture/7 -> myMux Fun5/5(u5)
  Input Capture/5 -> myMux Fun5/4(u4)
  Input Capture/4 -> myMux Fun5/3(u3)
  Input Capture/3 -> myMux Fun5/2(u2)
  Input Capture/2 -> myMux Fun5/1(u1)
  myMux Fun1/1(y) -> Voltage/Current Sensor/1
  Input Capture/6 -> Data Type Conversion2/1
  Input Capture/1 -> Data Type Conversion3/1
  2 sec  tau/1(Out1) -> Data Type Conversion1/1
  2 sec  tau1/1(Out1) -> Data Type Conversion4/1
  Data Type Conversion1/1 -> myMux Fun1/1(u1)
  Data Type Conversion4/1 -> myMux Fun1/2(u2)
  Data Type Conversion2/1 -> 2 sec  tau/1(In1)
  Data Type Conversion3/1 -> 2 sec  tau1/1(In1)

== system controlMCUSlugsMKIINewNav/Trim Vals/Convert to Microseconds  ==
  IC : Inport
  Convert to  Microseconds : Gain  Gain=0.2
  Data Type Conversion : DataTypeConversion  OutDataTypeStr=uint16
  uS : Outport
  wires:
  Convert to  Microseconds/1 -> Data Type Conversion/1
  IC/1 -> Convert to  Microseconds/1
  Data Type Conversion/1 -> uS/1

== system controlMCUSlugsMKIINewNav/Trim Vals/Detect Transition High to Low ==
  Switch : Inport
  IC1 : InitialCondition  Value=0
  Logical Operator : Logic  Operator=NOT  AllPortsSameDT=off  OutDataTypeStr=boolean
  Subsystem : Subsystem
  Transition : Outport
  wires:
  Switch/1 -> Logical Operator/1
  IC1/1 -> Subsystem/1(WP Fly)
  Logical Operator/1 -> IC1/1
  Subsystem/1(Just Enab) -> Transition/1

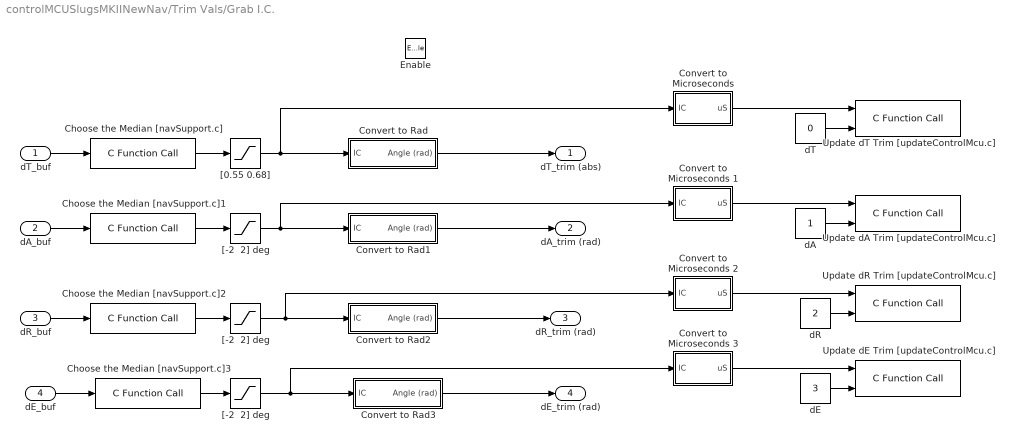
== system controlMCUSlugsMKIINewNav/Trim Vals/Grab I.C. ==
  dT_buf : Inport
  dA_buf : Inport  Port=2
  dR_buf : Inport  Port=3
  dE_buf : Inport  Port=4
  Enable : EnablePort
  Choose the Median [navSupport.c]{,1..3} (4 alike) : dsPICdrivers/OTHERS/C Function Call  Tag=dsPIC_dsPIC_CFunctionCall  FctUpdate=Output Function  fctName='meanFilter5'  INPUT_SIZE=7  INPUT1=uint16  INPUT2=--  INPUT3=--  OUTPUT_SIZE=1  OUTPUT1=uint16  SampleTime=.01  InputType=[ 4 ]  OutputType=[ 4 ]  FctDeclaration=extern uint16_T meanFilter5(uint16_T* u1);  FctCall=%y1 = meanFilter5(*%u1);  OrderingInOutPopup=None  FctStart=None  FctStart_Name=Init_onlyOnce  FctStart_Declaration=inline extern void Init_onlyOnce();  FctStart_Call=Init_onlyOnce();  FctInit=None  FctInit_Name=Init_Reset  FctInit_Declaration=inline extern void Init_Reset();  FctInit_Call=Init_Reset();  PinDigitalInput=[]  PinDigitalOutput=[]  AnalogueInput=[]
  "Convert to Microseconds " : Subsystem
  Convert to Microseconds 1 : Subsystem
  Convert to Microseconds 2 : Subsystem
  Convert to Microseconds 3 : Subsystem
  Convert to Rad : Subsystem  mask{slopem=mICdt, interceptb=bICdt}
      mask prompts: slopem "Slope"; interceptb "Intercept"
  Convert to Rad1 : Subsystem  mask{slopem=mICda, interceptb=bICda}
      mask prompts: slopem "Slope"; interceptb "Intercept"
  Convert to Rad2 : Subsystem  mask{slopem=mICdr, interceptb=bICdr}
      mask prompts: slopem "Slope"; interceptb "Intercept"
  Convert to Rad3 : Subsystem  mask{slopem=mICde, interceptb=bICde}
      mask prompts: slopem "Slope"; interceptb "Intercept"
  Update dA Trim [updateControlMcu.c] : dsPICdrivers/OTHERS/C Function Call  Tag=dsPIC_dsPIC_CFunctionCall  FctUpdate=Output Function  fctName='updatePWMTrim'  INPUT_SIZE=1  INPUT1=uint16  INPUT2=uint8  INPUT3=--  OUTPUT_SIZE=1  OUTPUT1=--  SampleTime=-1  InputType=[ 4 2 ]  OutputType=[ ]  FctDeclaration=extern void updatePWMTrim(uint16_T u1, uint8_T u2);  FctCall=updatePWMTrim(%u1, %u2);  OrderingInOutPopup=None  FctStart=None  FctStart_Name=Init_onlyOnce  FctStart_Declaration=inline extern void Init_onlyOnce();  FctStart_Call=Init_onlyOnce();  FctInit=None  FctInit_Name=Init_Reset  FctInit_Declaration=inline extern void Init_Reset();  FctInit_Call=Init_Reset();  PinDigitalInput=[]  PinDigitalOutput=[]  AnalogueInput=[]
  Update dE Trim [updateControlMcu.c] : dsPICdrivers/OTHERS/C Function Call  Tag=dsPIC_dsPIC_CFunctionCall  FctUpdate=Output Function  fctName='updatePWMTrim'  INPUT_SIZE=1  INPUT1=uint16  INPUT2=uint8  INPUT3=--  OUTPUT_SIZE=1  OUTPUT1=--  SampleTime=-1  InputType=[ 4 2 ]  OutputType=[ ]  FctDeclaration=extern void updatePWMTrim(uint16_T u1, uint8_T u2);  FctCall=updatePWMTrim(%u1, %u2);  OrderingInOutPopup=None  FctStart=None  FctStart_Name=Init_onlyOnce  FctStart_Declaration=inline extern void Init_onlyOnce();  FctStart_Call=Init_onlyOnce();  FctInit=None  FctInit_Name=Init_Reset  FctInit_Declaration=inline extern void Init_Reset();  FctInit_Call=Init_Reset();  PinDigitalInput=[]  PinDigitalOutput=[]  AnalogueInput=[]
  Update dR Trim [updateControlMcu.c] : dsPICdrivers/OTHERS/C Function Call  Tag=dsPIC_dsPIC_CFunctionCall  FctUpdate=Output Function  fctName='updatePWMTrim'  INPUT_SIZE=1  INPUT1=uint16  INPUT2=uint8  INPUT3=--  OUTPUT_SIZE=1  OUTPUT1=--  SampleTime=-1  InputType=[ 4 2 ]  OutputType=[ ]  FctDeclaration=extern void updatePWMTrim(uint16_T u1, uint8_T u2);  FctCall=updatePWMTrim(%u1, %u2);  OrderingInOutPopup=None  FctStart=None  FctStart_Name=Init_onlyOnce  FctStart_Declaration=inline extern void Init_onlyOnce();  FctStart_Call=Init_onlyOnce();  FctInit=None  FctInit_Name=Init_Reset  FctInit_Declaration=inline extern void Init_Reset();  FctInit_Call=Init_Reset();  PinDigitalInput=[]  PinDigitalOutput=[]  AnalogueInput=[]
  Update dT Trim [updateControlMcu.c] : dsPICdrivers/OTHERS/C Function Call  Tag=dsPIC_dsPIC_CFunctionCall  FctUpdate=Output Function  fctName='updatePWMTrim'  INPUT_SIZE=1  INPUT1=uint16  INPUT2=uint8  INPUT3=--  OUTPUT_SIZE=1  OUTPUT1=--  SampleTime=-1  InputType=[ 4 2 ]  OutputType=[ ]  FctDeclaration=extern void updatePWMTrim(uint16_T u1, uint8_T u2);  FctCall=updatePWMTrim(%u1, %u2);  OrderingInOutPopup=None  FctStart=None  FctStart_Name=Init_onlyOnce  FctStart_Declaration=inline extern void Init_onlyOnce();  FctStart_Call=Init_onlyOnce();  FctInit=None  FctInit_Name=Init_Reset  FctInit_Declaration=inline extern void Init_Reset();  FctInit_Call=Init_Reset();  PinDigitalInput=[]  PinDigitalOutput=[]  AnalogueInput=[]
  "[-2  2] deg" : Saturate  UpperLimit=daTrimMax  LowerLimit=daTrimMin
  "[-2  2] deg " : Saturate  UpperLimit=drTrimMax  LowerLimit=drTrimMin
  "[-2  2] deg  " : Saturate  UpperLimit=deTrimMax  LowerLimit=deTrimMin
  "[0.55 0.68]" : Saturate  UpperLimit=dtTrimMax  LowerLimit=dtTrimMin
  dA : Constant  OutDataTypeStr=uint8
  dE : Constant  Value=3  OutDataTypeStr=uint8
  dR : Constant  Value=2  OutDataTypeStr=uint8
  dT : Constant  Value=0  OutDataTypeStr=uint8
  dT_trim (abs) : Outport
  dA_trim (rad) : Outport  Port=2
  dR_trim (rad) : Outport  Port=3
  dE_trim (rad) : Outport  Port=4
  wires:
  Convert to Rad/1(Angle (rad)) -> dT_trim (abs)/1
  Convert to Rad2/1(Angle (rad)) -> dR_trim (rad)/1
  Convert to Rad3/1(Angle (rad)) -> dE_trim (rad)/1
  Choose the Median [navSupport.c]/1 -> "[0.55 0.68]"/1
  Choose the Median [navSupport.c]1/1 -> "[-2  2] deg"/1
  Choose the Median [navSupport.c]2/1 -> "[-2  2] deg "/1
  Choose the Median [navSupport.c]3/1 -> "[-2  2] deg  "/1
  dT_buf/1 -> Choose the Median [navSupport.c]/1
  dA_buf/1 -> Choose the Median [navSupport.c]1/1
  dR_buf/1 -> Choose the Median [navSupport.c]2/1
  dE_buf/1 -> Choose the Median [navSupport.c]3/1
  dR/1 -> Update dR Trim [updateControlMcu.c]/2
  dE/1 -> Update dE Trim [updateControlMcu.c]/2
  dT/1 -> Update dT Trim [updateControlMcu.c]/2
  dA/1 -> Update dA Trim [updateControlMcu.c]/2
  "Convert to Microseconds "/1(uS) -> Update dT Trim [updateControlMcu.c]/1
  Convert to Microseconds 1/1(uS) -> Update dA Trim [updateControlMcu.c]/1
  Convert to Microseconds 2/1(uS) -> Update dR Trim [updateControlMcu.c]/1
  Convert to Microseconds 3/1(uS) -> Update dE Trim [updateControlMcu.c]/1
  "[0.55 0.68]"/1 -> Convert to Rad/1(IC), "Convert to Microseconds "/1(IC)
  "[-2  2] deg"/1 -> Convert to Rad1/1(IC), Convert to Microseconds 1/1(IC)
  "[-2  2] deg "/1 -> Convert to Rad2/1(IC), Convert to Microseconds 2/1(IC)
  "[-2  2] deg  "/1 -> Convert to Rad3/1(IC), Convert to Microseconds 3/1(IC)
  Convert to Rad1/1(Angle (rad)) -> dA_trim (rad)/1

== system controlMCUSlugsMKIINewNav/Trim Vals/Mean Filter the Transition ==
  Failsafe : Inport
  Buffer Failsafe Channel : MATLAB Function  TreatAsAtomicUnit=on
  Choose the Median [navSupport.c] : dsPICdrivers/OTHERS/C Function Call  Tag=dsPIC_dsPIC_CFunctionCall  FctUpdate=Output Function  fctName='meanFilter5'  INPUT_SIZE=7  INPUT1=uint16  INPUT2=--  INPUT3=--  OUTPUT_SIZE=1  OUTPUT1=uint16  SampleTime=.01  InputType=[ 4 ]  OutputType=[ 4 ]  FctDeclaration=extern uint16_T meanFilter5(uint16_T* u1);  FctCall=%y1 = meanFilter5(*%u1);  OrderingInOutPopup=None  FctStart=None  FctStart_Name=Init_onlyOnce  FctStart_Declaration=inline extern void Init_onlyOnce();  FctStart_Call=Init_onlyOnce();  FctInit=None  FctInit_Name=Init_Reset  FctInit_Declaration=inline extern void Init_Reset();  FctInit_Call=Init_Reset();  PinDigitalInput=[]  PinDigitalOutput=[]  AnalogueInput=[]
  filtered : Outport
  wires:
  Buffer Failsafe Channel/1(history) -> Choose the Median [navSupport.c]/1
  Failsafe/1 -> Buffer Failsafe Channel/1(latest)
  Choose the Median [navSupport.c]/1 -> filtered/1

== system controlMCUSlugsMKIINewNav/Update PWM Commands and Send Telemetry/Convert to Microseconds ==
  PWM : Inport
  Convert to  Microseconds : Gain  Gain=0.4
  Data Type Conversion : DataTypeConversion  OutDataTypeStr=uint16
  uS : Outport
  wires:
  Data Type Conversion/1 -> uS/1
  PWM/1 -> Convert to  Microseconds/1
  Convert to  Microseconds/1 -> Data Type Conversion/1

== system controlMCUSlugsMKIINewNav/Update PWM Commands and Send Telemetry/Generate PWM Signals Based on the Control Type ==
  note: Navigation Modes:
      | 2 -> PT
      | 3 -> Waypoint
      | 4 -> Mid Level
      | 8-> Sel PT
      | 9-> ISR
      | 10 -> Line Patrol
  PWM(rad) : Inport
  Pilot Console (IC) : Inport  Port=2
  isManual? : Inport  Port=3
  Nav Mode : Inport  Port=4
  Data Type Conversion : DataTypeConversion  OutDataTypeStr=uint16
  If : If  NumInputs=2  IfExpression=u2 == 1  ElseIfExpressions=((u1 == 3) | (u1 == 4) | (u1 == 9) | (u1 == 10)), u1 == 2, u1 == 8  ShowElse=off  SampleTime=.01
  If  Control Type Is Manual : Subsystem  TreatAsAtomicUnit=on
  If  Control Type Is Passthrough : Subsystem  TreatAsAtomicUnit=on
  If  Control Type Is Selective Passthrough : Subsystem  TreatAsAtomicUnit=on
  "If  Control Type Is Wp, ISR, LP or  Mid Lvl Cmds" : Subsystem  TreatAsAtomicUnit=on
  Merge : Merge  Inputs=4
  PWM : Outport
  wires:
  If/1 -> If  Control Type Is Manual/Action
  If/2 -> "If  Control Type Is Wp, ISR, LP or  Mid Lvl Cmds"/Action
  If/3 -> If  Control Type Is Passthrough/Action
  If/4 -> If  Control Type Is Selective Passthrough/Action
  If  Control Type Is Manual/1(PWM) -> Merge/1
  "If  Control Type Is Wp, ISR, LP or  Mid Lvl Cmds"/1(PWM (abs)) -> Merge/2
  If  Control Type Is Passthrough/1(PWM (abs)) -> Merge/3
  If  Control Type Is Selective Passthrough/1(PWM) -> Merge/4
  PWM(rad)/1 -> "If  Control Type Is Wp, ISR, LP or  Mid Lvl Cmds"/1(PWM(rad)), If  Control Type Is Selective Passthrough/1(PWM(rad))
  Pilot Console (IC)/1 -> If  Control Type Is Manual/1(Pilot (IC)), If  Control Type Is Passthrough/1(Pilot (IC)), If  Control Type Is Selective Passthrough/2(Pilot (IC))
  Nav Mode/1 -> If/1
  Merge/1 -> Data Type Conversion/1
  Data Type Conversion/1 -> PWM/1
  isManual?/1 -> If/2
